simulink model "noisefilter"  (Simulink 7.7)
settings: Solver=ode45  StartTime=0.0  StopTime=1000  RelTol=1e-3
libraries: commnoisgen2 x1
settings Model: Creator=kevin  LastModifiedBy=kevin

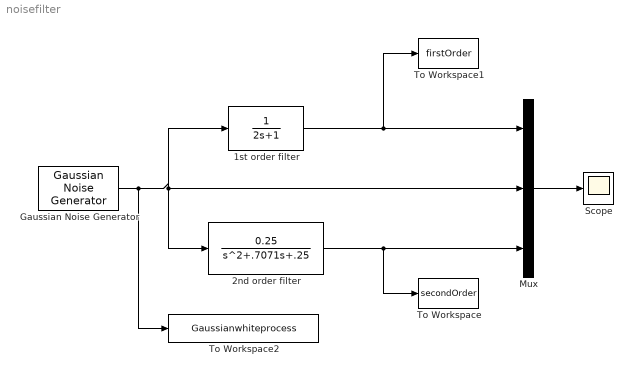
== system noisefilter ==
  1st order filter : TransferFcn  Denominator=[2 1]
  2nd order filter : TransferFcn  Numerator=[0.25]  Denominator=[1 .7071 .25]
  Gaussian Noise Generator : commnoisgen2/Gaussian Noise Generator  SystemSampleTime=-1  m=0  d=1  s=41  Ts=.1  frameBased=off  sampPerFrame=1  orient=off  outDataType=double
  Mux : Mux  Inputs=3
  Scope : Scope
  To Workspace : ToWorkspace  VariableName=secondOrder  SampleTime=-1  SaveFormat=Array
  To Workspace1 : ToWorkspace  VariableName=firstOrder  SampleTime=-1  SaveFormat=Array
  To Workspace2 : ToWorkspace  VariableName=Gaussianwhiteprocess  SampleTime=-1  SaveFormat=Array
  wires:
  Mux/1 -> Scope/1
  Gaussian Noise Generator/1 -> 1st order filter/1, 2nd order filter/1, Mux/2, To Workspace2/1
  2nd order filter/1 -> Mux/3, To Workspace/1
  1st order filter/1 -> Mux/1, To Workspace1/1
